simulink model "Full_model"  (R2019b)
settings: Solver=VariableStepAuto  StartTime=0.0  StopTime=150  RelTol=1e-3
model workspace: external: MATLAB File C:\Users\Techboard IITG\Downloads\Simscape4\Full_assem_DataFile.m (data not in the file)
undefined symbols (not defined in the file): _Default_sldprt, apx, ch_app, ch_cyc, cpz, L1, L2, L2rz, L2xf, L2yf, L2zf, l_app, max_avel, max_tvel, smiData, stand, TH1_ec_i, TH1_f, TH1_i, TH1_i_r, TH1_ri, TH2_ec_i, TH2_f, TH2_i, TH2_i_r, TH2_ri, TH3_f, TH3_i, TH3_ri, TH4_f, TH4_i, TH4_ri, time_ch_app, time_if, time_plug, time_ri, time_zchapp_down, time_zchapp_up, X, xp_dist, xp_vel, xpf_i, Y, yp_dist, yp_vel, ypf_i, Z, z_chapp, Z_i, zp_dist, zp_vel, zpf_i
libraries: simulink x68, fl_lib x36, sm_lib x22, nesl_utility x21, ee_lib x12
(part 2 of 3)

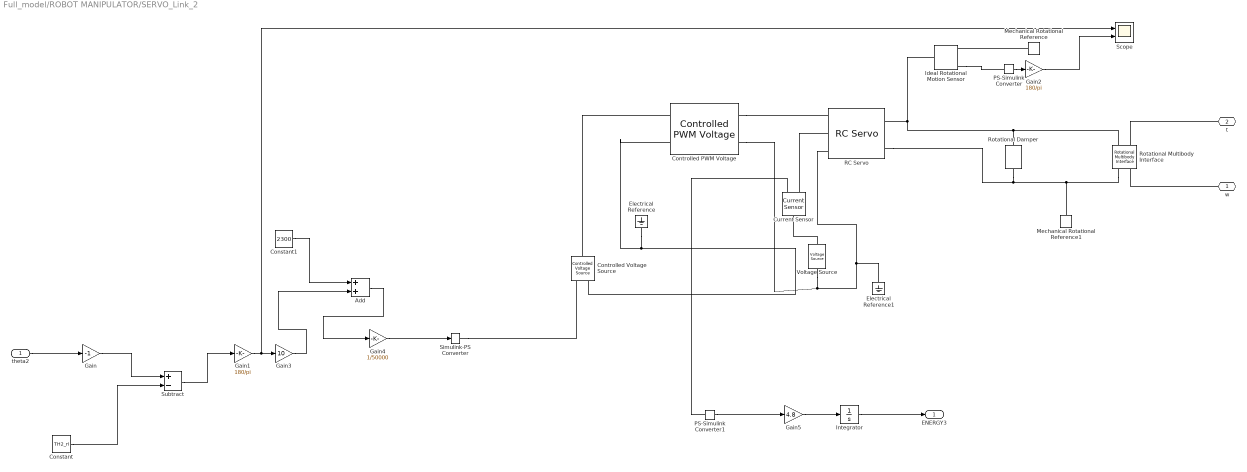
== system Full_model/ROBOT MANIPULATOR/SERVO_Link_2 ==
  theta2 : Inport
  Add : Sum
  Constant : Constant  Value=TH2_ri
  Constant1 : Constant  Value=2300
  Controlled PWM Voltage : ee_lib/Integrated Circuits/Controlled PWM Voltage  F=20 Hz  TD=0 s  pulse_width_offset=0 s  pulse_min=0 s  pwm_or_av=1  event_type=1  sample_time=1e-6 s  Vmin=0 V  Vmax=1 V  Vm=5 V  u_min=0  u_max=1
  Controlled Voltage Source : fl_lib/Electrical/Electrical Sources/Controlled Voltage Source
  Current Sensor : fl_lib/Electrical/Electrical Sensors/Current Sensor
      settings: SourceProductBaseCode=PW,SS,VE
  Electrical Reference : fl_lib/Electrical/Electrical Elements/Electrical Reference
  Electrical Reference1 : fl_lib/Electrical/Electrical Elements/Electrical Reference
  Gain : Gain  Gain=-1
  Gain1 : Gain  Gain=180/pi
  Gain2 : Gain  Gain=180/pi
  Gain3 : Gain  Gain=10
  Gain4 : Gain  Gain=1/50000
  Gain5 : Gain  Gain=4.8
  Ideal Rotational Motion Sensor : fl_lib/Mechanical/Mechanical Sensors/Ideal Rotational Motion Sensor  wrap_angle=simscape.enum.onoff.off  offset=0 rad
      settings: SourceProductBaseCode=PW,SS,VE
  Integrator : Integrator
  Mechanical Rotational Reference : fl_lib/Mechanical/Rotational Elements/Mechanical Rotational Reference
      settings: SourceProductBaseCode=PW,SS,VE
  Mechanical Rotational Reference1 : fl_lib/Mechanical/Rotational Elements/Mechanical Rotational Reference
  PS-Simulink Converter : nesl_utility/PS-Simulink Converter  PhysicalDomain=network_engine_domain  SubClassName=ps_output  LeftPortType=input  RightPortType=output  PseudoPeriodic=off  Frequencies=[]  VectorFormat=inherit  Unit=inherit  AffineConversion=off
      settings: SourceProductBaseCode=SS,PW,VE
  PS-Simulink Converter1 : nesl_utility/PS-Simulink Converter  PhysicalDomain=network_engine_domain  SubClassName=ps_output  LeftPortType=input  RightPortType=output  PseudoPeriodic=off  Frequencies=[]  VectorFormat=inherit  Unit=inherit  AffineConversion=off
      settings: SourceProductBaseCode=SS,PW,VE
  RC Servo : ee_lib/Electromechanical/Brushed Motors/RC Servo  stall_torque=25 kg*cm  time_60=0.28 s  nominal_voltage=4.8 V  rotational_range=[-90, 270] deg  pulse_width_range=[500, 4100] us  threshold=3 V  R_s=18 kOhm  resolution=0.1 deg  angle_meas_error=0 deg  backdrive_torque=0.5 kg*cm  ratio=320  inertia=0.01 g*cm^2  endstop_angles=[-90, 270] deg  endstop_stiffness=1e6 N*m/rad  endstop_damping=0.01 N*m/(rad/s)  enable_faults=0  fault_action=1  fault_type=1  enable_temporal_fault=0  t_fault=1 s  enable_behavioral_fault=0  max_permissible_current=1 A  t_fail_on_current=1 s  angle_specify=off  angle_priority=High  angle=90 deg  angle_nominal_specify=off  angle_nominal_unit=deg  angle_nominal_value=1  w_specify=off  w_priority=High  w=0 deg/s  w_nominal_specify=off  w_nominal_unit=deg/s  w_nominal_value=1  torque_specify=off  torque_priority=None  torque=0 N*m  torque_nominal_specify=off  torque_nominal_unit=N*m  torque_nominal_value=1  pulse_width_specify=off  pulse_width_priority=Low  pulse_width=1.5 ms  i_specify=off  i_priority=None  i=0 A  i_nominal_specify=off  i_nominal_unit=A  i_nominal_value=1  i_s_specify=off  i_s_priority=None  i_s=0 A  i_s_nominal_specify=off  i_s_nominal_unit=A  i_s_nominal_value=1  motor_torque_specify=off  motor_torque_priority=None  motor_torque=0 N*m  motor_torque_nominal_specify=off  motor_torque_nominal_unit=N*m  motor_torque_nominal_value=1  power_dissipated_specify=off  power_dissipated_priority=None  power_dissipated=0 W  power_dissipated_nominal_specify=off  power_dissipated_nominal_unit=W  power_dissipated_nominal_value=1  angle_demand_specify=off  angle_demand_priority=None  angle_demand=90 deg  angle_demand_nominal_specify=off  angle_demand_nominal_unit=deg  angle_demand_nominal_value=1  faulted_specify=off  faulted_priority=None  faulted=0  faulted_nominal_specify=off  faulted_nominal_unit=1  faulted_nominal_value=1
      settings: SourceProductBaseCode=PS  InternalSimscapePortConfiguration="{\"Bottom\":[],\"Left\":[{\"id\":\"s\",\"label\":\"s\",\"type\":\"foundation.electrical.electrical\"},{\"id\":\"p\",\"label\":\"+\",\"type\":\"foundation.electrical.electrical\"},{\"id\":\"n\",\"label\":\"-\",\"type\":\"foundation.electrical.electrical\"}],\"Right\":[{\"id\":\"R\",\"label\":\"R\",\"type\":\"foundation.mechanical.rotational.rotational\"},{\"id\":\"C\",\"label\":\"C\",\"type\":\"foundation.mechanical.rotational.rotational\"}],\"Top\":[]}"
  Rotational Damper : fl_lib/Mechanical/Rotational Elements/Rotational Damper  D=15 N*m*s/rad  w_specify=off  w_priority=None  w=0 rad/s  w_nominal_specify=off  w_nominal_unit=rad/s  w_nominal_value=1  t_specify=off  t_priority=None  t=0 N*m  t_nominal_specify=off  t_nominal_unit=N*m  t_nominal_value=1
      settings: SourceProductBaseCode=PW,SS,VE
  Rotational Multibody Interface : fl_lib/Mechanical/Multibody Interfaces/Rotational Multibody Interface
      settings: SourceProductBaseCode=PW,SS,VE
  Scope : Scope  NumInputPorts=2
  Simulink-PS Converter : nesl_utility/Simulink-PS Converter  PhysicalDomain=network_engine_domain  SubClassName=ps_input  LeftPortType=input  RightPortType=output  PseudoPeriodic=off  Frequencies=[]  NoiseDistribution=none  NoiseParameters=[]  Unit=1  AffineConversion=off  FilteringAndDerivatives=provide  SimscapeFilterOrder=1  InputFilterTimeConstant=0.001  UdotUserProvided=0
      settings: SourceProductBaseCode=PW,SS
  Subtract : Sum  Inputs=+-
  Voltage Source : ee_lib/Sources/Voltage Source  dc_voltage=4.8 V  ac_voltage=0 V  ac_shift=0 rad  ac_frequency=60 Hz  noise_mode=0  PSD=0 V^2/Hz  repeatability=1  auto_seed=2715962282  user_seed=0  sample_time=1e-3 s  i_specify=off  i_priority=None  i=0 A  i_nominal_specify=off  i_nominal_unit=A  i_nominal_value=1  v_specify=off  v_priority=None  v=0 V  v_nominal_specify=off  v_nominal_unit=V  v_nominal_value=1
  w : PMIOPort  Side=Right
  t : PMIOPort  Port=2  Side=Left
  ENERGY3 : Outport
  wires:
  Add/1 -> Gain4/1
  Gain4/1 -> Simulink-PS Converter/1
  Gain1/1 -> Scope/1, Gain3/1
  Gain3/1 -> Add/2
  Constant1/1 -> Add/1
  theta2/1 -> Gain/1
  PS-Simulink Converter/1 -> Gain2/1
  Gain/1 -> Subtract/1
  Constant/1 -> Subtract/2
  Subtract/1 -> Gain1/1
  PS-Simulink Converter1/1 -> Gain5/1
  Gain5/1 -> Integrator/1
  Integrator/1 -> ENERGY3/1
  Gain2/1 -> Scope/2
  connections:
  Rotational Damper/RConn1 -- Rotational Multibody Interface/RConn2 -- Mechanical Rotational Reference1/LConn1 -- RC Servo/RConn2
  Voltage Source/RConn1 -- Electrical Reference1/LConn1 -- RC Servo/LConn3 -- Controlled PWM Voltage/RConn2
  Electrical Reference/LConn1 -- Controlled Voltage Source/RConn2 -- Controlled PWM Voltage/LConn2
  Controlled Voltage Source/LConn1 -- Controlled PWM Voltage/LConn1
  Rotational Multibody Interface/LConn2 -- Rotational Damper/LConn1 -- Ideal Rotational Motion Sensor/LConn1 -- RC Servo/RConn1
  Controlled PWM Voltage/RConn1 -- RC Servo/LConn1
  Simulink-PS Converter/RConn1 -- Controlled Voltage Source/RConn1
  t/RConn1 -- Rotational Multibody Interface/LConn1
  Ideal Rotational Motion Sensor/RConn3 -- PS-Simulink Converter/LConn1
  Mechanical Rotational Reference/LConn1 -- Ideal Rotational Motion Sensor/RConn1
  w/RConn1 -- Rotational Multibody Interface/RConn1
  Voltage Source/LConn1 -- Current Sensor/LConn1
  Current Sensor/RConn2 -- RC Servo/LConn2
  Current Sensor/RConn1 -- PS-Simulink Converter1/LConn1

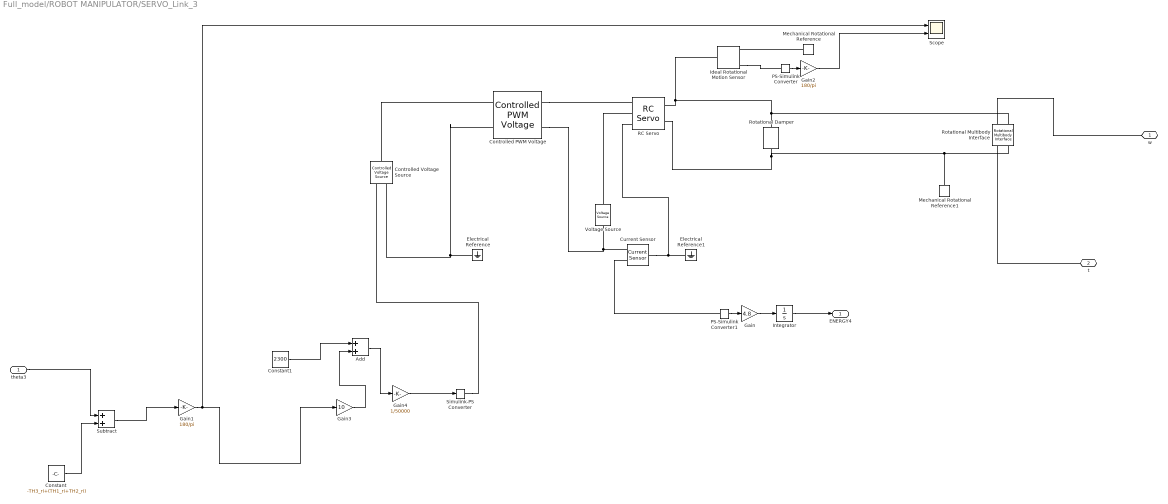
== system Full_model/ROBOT MANIPULATOR/SERVO_Link_3 ==
  theta3 : Inport
  Add : Sum
  Constant : Constant  Value=-TH3_ri+(TH1_ri+TH2_ri)
  Constant1 : Constant  Value=2300
  Controlled PWM Voltage : ee_lib/Integrated Circuits/Controlled PWM Voltage  F=20 Hz  TD=0 s  pulse_width_offset=0 s  pulse_min=0 s  pwm_or_av=1  event_type=1  sample_time=1e-6 s  Vmin=0 V  Vmax=1 V  Vm=5 V  u_min=0  u_max=1
  Controlled Voltage Source : fl_lib/Electrical/Electrical Sources/Controlled Voltage Source
  Current Sensor : fl_lib/Electrical/Electrical Sensors/Current Sensor
      settings: SourceProductBaseCode=PW,SS,VE
  Electrical Reference : fl_lib/Electrical/Electrical Elements/Electrical Reference
  Electrical Reference1 : fl_lib/Electrical/Electrical Elements/Electrical Reference
  Gain : Gain  Gain=4.8
  Gain1 : Gain  Gain=180/pi
  Gain2 : Gain  Gain=180/pi
  Gain3 : Gain  Gain=10
  Gain4 : Gain  Gain=1/50000
  Ideal Rotational Motion Sensor : fl_lib/Mechanical/Mechanical Sensors/Ideal Rotational Motion Sensor  wrap_angle=simscape.enum.onoff.off  offset=0 rad
      settings: SourceProductBaseCode=PW,SS,VE
  Integrator : Integrator
  Mechanical Rotational Reference : fl_lib/Mechanical/Rotational Elements/Mechanical Rotational Reference
      settings: SourceProductBaseCode=PW,SS,VE
  Mechanical Rotational Reference1 : fl_lib/Mechanical/Rotational Elements/Mechanical Rotational Reference
  PS-Simulink Converter : nesl_utility/PS-Simulink Converter  PhysicalDomain=network_engine_domain  SubClassName=ps_output  LeftPortType=input  RightPortType=output  PseudoPeriodic=off  Frequencies=[]  VectorFormat=inherit  Unit=inherit  AffineConversion=off
      settings: SourceProductBaseCode=SS,PW,VE
  PS-Simulink Converter1 : nesl_utility/PS-Simulink Converter  PhysicalDomain=network_engine_domain  SubClassName=ps_output  LeftPortType=input  RightPortType=output  PseudoPeriodic=off  Frequencies=[]  VectorFormat=inherit  Unit=inherit  AffineConversion=off
      settings: SourceProductBaseCode=SS,PW,VE
  RC Servo : ee_lib/Electromechanical/Brushed Motors/RC Servo  stall_torque=25 kg*cm  time_60=0.28 s  nominal_voltage=4.8 V  rotational_range=[-90,270] deg  pulse_width_range=[500, 4100] us  threshold=3 V  R_s=18 kOhm  resolution=0.1 deg  angle_meas_error=0 deg  backdrive_torque=0.5 kg*cm  ratio=320  inertia=0.01 g*cm^2  endstop_angles=[-90, 270] deg  endstop_stiffness=1e6 N*m/rad  endstop_damping=0.01 N*m/(rad/s)  enable_faults=0  fault_action=1  fault_type=1  enable_temporal_fault=0  t_fault=1 s  enable_behavioral_fault=0  max_permissible_current=1 A  t_fail_on_current=1 s  angle_specify=off  angle_priority=High  angle=90 deg  angle_nominal_specify=off  angle_nominal_unit=deg  angle_nominal_value=1  w_specify=off  w_priority=High  w=0 deg/s  w_nominal_specify=off  w_nominal_unit=deg/s  w_nominal_value=1  torque_specify=off  torque_priority=None  torque=0 N*m  torque_nominal_specify=off  torque_nominal_unit=N*m  torque_nominal_value=1  pulse_width_specify=off  pulse_width_priority=Low  pulse_width=1.5 ms  i_specify=off  i_priority=None  i=0 A  i_nominal_specify=off  i_nominal_unit=A  i_nominal_value=1  i_s_specify=off  i_s_priority=None  i_s=0 A  i_s_nominal_specify=off  i_s_nominal_unit=A  i_s_nominal_value=1  motor_torque_specify=off  motor_torque_priority=None  motor_torque=0 N*m  motor_torque_nominal_specify=off  motor_torque_nominal_unit=N*m  motor_torque_nominal_value=1  power_dissipated_specify=off  power_dissipated_priority=None  power_dissipated=0 W  power_dissipated_nominal_specify=off  power_dissipated_nominal_unit=W  power_dissipated_nominal_value=1  angle_demand_specify=off  angle_demand_priority=None  angle_demand=90 deg  angle_demand_nominal_specify=off  angle_demand_nominal_unit=deg  angle_demand_nominal_value=1  faulted_specify=off  faulted_priority=None  faulted=0  faulted_nominal_specify=off  faulted_nominal_unit=1  faulted_nominal_value=1
      settings: SourceProductBaseCode=PS  InternalSimscapePortConfiguration="{\"Bottom\":[],\"Left\":[{\"id\":\"s\",\"label\":\"s\",\"type\":\"foundation.electrical.electrical\"},{\"id\":\"p\",\"label\":\"+\",\"type\":\"foundation.electrical.electrical\"},{\"id\":\"n\",\"label\":\"-\",\"type\":\"foundation.electrical.electrical\"}],\"Right\":[{\"id\":\"R\",\"label\":\"R\",\"type\":\"foundation.mechanical.rotational.rotational\"},{\"id\":\"C\",\"label\":\"C\",\"type\":\"foundation.mechanical.rotational.rotational\"}],\"Top\":[]}"
  Rotational Damper : fl_lib/Mechanical/Rotational Elements/Rotational Damper  D=15 N*m*s/rad  w_specify=off  w_priority=None  w=0 rad/s  w_nominal_specify=off  w_nominal_unit=rad/s  w_nominal_value=1  t_specify=off  t_priority=None  t=0 N*m  t_nominal_specify=off  t_nominal_unit=N*m  t_nominal_value=1
      settings: SourceProductBaseCode=PW,SS,VE
  Rotational Multibody Interface : fl_lib/Mechanical/Multibody Interfaces/Rotational Multibody Interface
      settings: SourceProductBaseCode=PW,SS,VE
  Scope : Scope  NumInputPorts=2
  Simulink-PS Converter : nesl_utility/Simulink-PS Converter  PhysicalDomain=network_engine_domain  SubClassName=ps_input  LeftPortType=input  RightPortType=output  PseudoPeriodic=off  Frequencies=[]  NoiseDistribution=none  NoiseParameters=[]  Unit=1  AffineConversion=off  FilteringAndDerivatives=provide  SimscapeFilterOrder=1  InputFilterTimeConstant=0.001  UdotUserProvided=0
      settings: SourceProductBaseCode=PW,SS
  Subtract : Sum
  Voltage Source : ee_lib/Sources/Voltage Source  dc_voltage=4.8 V  ac_voltage=0 V  ac_shift=0 rad  ac_frequency=60 Hz  noise_mode=0  PSD=0 V^2/Hz  repeatability=1  auto_seed=418932850  user_seed=0  sample_time=1e-3 s  i_specify=off  i_priority=None  i=0 A  i_nominal_specify=off  i_nominal_unit=A  i_nominal_value=1  v_specify=off  v_priority=None  v=0 V  v_nominal_specify=off  v_nominal_unit=V  v_nominal_value=1
  w : PMIOPort  Side=Right
  t : PMIOPort  Port=2  Side=Left
  ENERGY4 : Outport
  wires:
  Add/1 -> Gain4/1
  Gain4/1 -> Simulink-PS Converter/1
  Gain3/1 -> Add/2
  Constant1/1 -> Add/1
  PS-Simulink Converter/1 -> Gain2/1
  theta3/1 -> Subtract/1
  Gain1/1 -> Scope/1, Gain3/1
  Constant/1 -> Subtract/2
  Subtract/1 -> Gain1/1
  Gain2/1 -> Scope/2
  PS-Simulink Converter1/1 -> Gain/1
  Gain/1 -> Integrator/1
  Integrator/1 -> ENERGY4/1
  connections:
  Rotational Damper/RConn1 -- RC Servo/RConn2 -- Mechanical Rotational Reference1/LConn1 -- Rotational Multibody Interface/LConn2
  Rotational Multibody Interface/RConn1 -- w/RConn1
  Electrical Reference1/LConn1 -- Current Sensor/LConn1 -- RC Servo/LConn3
  Electrical Reference/LConn1 -- Controlled PWM Voltage/LConn2 -- Controlled Voltage Source/RConn2
  Controlled Voltage Source/LConn1 -- Controlled PWM Voltage/LConn1
  Rotational Damper/LConn1 -- Ideal Rotational Motion Sensor/LConn1 -- RC Servo/RConn1 -- Rotational Multibody Interface/RConn2
  Voltage Source/LConn1 -- RC Servo/LConn2
  Controlled PWM Voltage/RConn1 -- RC Servo/LConn1
  Simulink-PS Converter/RConn1 -- Controlled Voltage Source/RConn1
  t/RConn1 -- Rotational Multibody Interface/LConn1
  Ideal Rotational Motion Sensor/RConn3 -- PS-Simulink Converter/LConn1
  Mechanical Rotational Reference/LConn1 -- Ideal Rotational Motion Sensor/RConn1
  Controlled PWM Voltage/RConn2 -- Current Sensor/RConn2 -- Voltage Source/RConn1
  Current Sensor/RConn1 -- PS-Simulink Converter1/LConn1

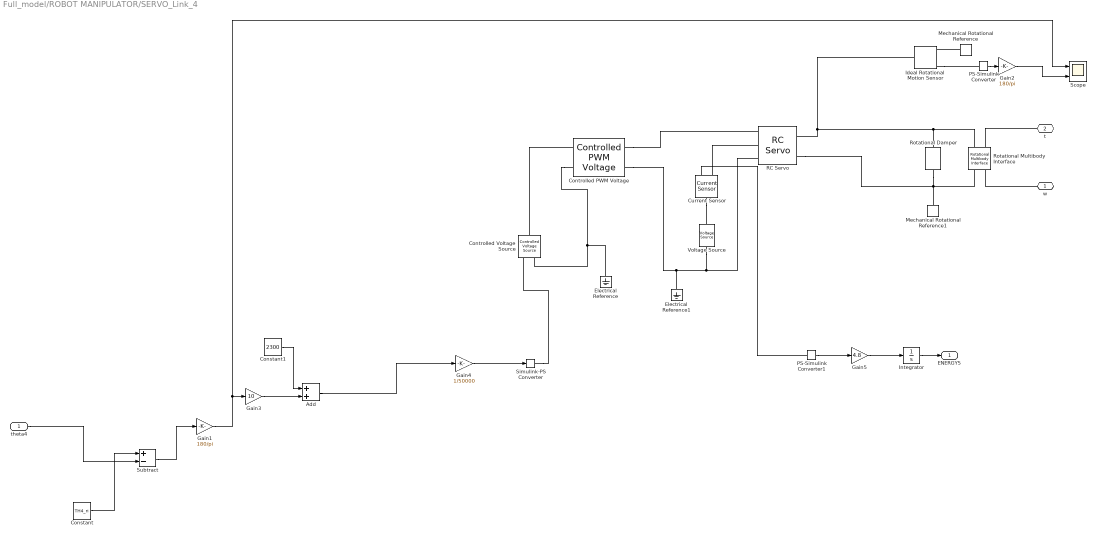
== system Full_model/ROBOT MANIPULATOR/SERVO_Link_4 ==
  theta4 : Inport
  Add : Sum
  Constant : Constant  Value=TH4_ri
  Constant1 : Constant  Value=2300
  Controlled PWM Voltage : ee_lib/Integrated Circuits/Controlled PWM Voltage  F=20 Hz  TD=0 s  pulse_width_offset=0 s  pulse_min=0 s  pwm_or_av=1  event_type=1  sample_time=1e-6 s  Vmin=0 V  Vmax=1 V  Vm=5 V  u_min=0  u_max=1
  Controlled Voltage Source : fl_lib/Electrical/Electrical Sources/Controlled Voltage Source
  Current Sensor : fl_lib/Electrical/Electrical Sensors/Current Sensor
      settings: SourceProductBaseCode=PW,SS,VE
  Electrical Reference : fl_lib/Electrical/Electrical Elements/Electrical Reference
  Electrical Reference1 : fl_lib/Electrical/Electrical Elements/Electrical Reference
  Gain1 : Gain  Gain=180/pi
  Gain2 : Gain  Gain=180/pi
  Gain3 : Gain  Gain=10
  Gain4 : Gain  Gain=1/50000
  Gain5 : Gain  Gain=4.8
  Ideal Rotational Motion Sensor : fl_lib/Mechanical/Mechanical Sensors/Ideal Rotational Motion Sensor  wrap_angle=simscape.enum.onoff.off  offset=0 rad
      settings: SourceProductBaseCode=PW,SS,VE
  Integrator : Integrator
  Mechanical Rotational Reference : fl_lib/Mechanical/Rotational Elements/Mechanical Rotational Reference
      settings: SourceProductBaseCode=PW,SS,VE
  Mechanical Rotational Reference1 : fl_lib/Mechanical/Rotational Elements/Mechanical Rotational Reference
  PS-Simulink Converter : nesl_utility/PS-Simulink Converter  PhysicalDomain=network_engine_domain  SubClassName=ps_output  LeftPortType=input  RightPortType=output  PseudoPeriodic=off  Frequencies=[]  VectorFormat=inherit  Unit=inherit  AffineConversion=off
      settings: SourceProductBaseCode=SS,PW,VE
  PS-Simulink Converter1 : nesl_utility/PS-Simulink Converter  PhysicalDomain=network_engine_domain  SubClassName=ps_output  LeftPortType=input  RightPortType=output  PseudoPeriodic=off  Frequencies=[]  VectorFormat=inherit  Unit=inherit  AffineConversion=off
      settings: SourceProductBaseCode=SS,PW,VE
  RC Servo : ee_lib/Electromechanical/Brushed Motors/RC Servo  stall_torque=25 kg*cm  time_60=0.28 s  nominal_voltage=4.8 V  rotational_range=[-90, 270] deg  pulse_width_range=[500, 4100] us  threshold=3 V  R_s=18 kOhm  resolution=0.1 deg  angle_meas_error=0 deg  backdrive_torque=0.5 kg*cm  ratio=320  inertia=0.01 g*cm^2  endstop_angles=[-90, 270] deg  endstop_stiffness=1e6 N*m/rad  endstop_damping=0.01 N*m/(rad/s)  enable_faults=0  fault_action=1  fault_type=1  enable_temporal_fault=0  t_fault=1 s  enable_behavioral_fault=0  max_permissible_current=1 A  t_fail_on_current=1 s  angle_specify=off  angle_priority=None  angle=5 deg  angle_nominal_specify=off  angle_nominal_unit=deg  angle_nominal_value=1  w_specify=off  w_priority=High  w=0 deg/s  w_nominal_specify=off  w_nominal_unit=deg/s  w_nominal_value=1  torque_specify=off  torque_priority=None  torque=0 N*m  torque_nominal_specify=off  torque_nominal_unit=N*m  torque_nominal_value=1  pulse_width_specify=off  pulse_width_priority=High  pulse_width=2 ms  i_specify=off  i_priority=None  i=0 A  i_nominal_specify=off  i_nominal_unit=A  i_nominal_value=1  i_s_specify=off  i_s_priority=None  i_s=0 A  i_s_nominal_specify=off  i_s_nominal_unit=A  i_s_nominal_value=1  motor_torque_specify=off  motor_torque_priority=None  motor_torque=0 N*m  motor_torque_nominal_specify=off  motor_torque_nominal_unit=N*m  motor_torque_nominal_value=1  power_dissipated_specify=off  power_dissipated_priority=None  power_dissipated=0 W  power_dissipated_nominal_specify=off  power_dissipated_nominal_unit=W  power_dissipated_nominal_value=1  angle_demand_specify=off  angle_demand_priority=None  angle_demand=90 deg  angle_demand_nominal_specify=off  angle_demand_nominal_unit=deg  angle_demand_nominal_value=1  faulted_specify=off  faulted_priority=None  faulted=0  faulted_nominal_specify=off  faulted_nominal_unit=1  faulted_nominal_value=1
      settings: SourceProductBaseCode=PS  InternalSimscapePortConfiguration="{\"Bottom\":[],\"Left\":[{\"id\":\"s\",\"label\":\"s\",\"type\":\"foundation.electrical.electrical\"},{\"id\":\"p\",\"label\":\"+\",\"type\":\"foundation.electrical.electrical\"},{\"id\":\"n\",\"label\":\"-\",\"type\":\"foundation.electrical.electrical\"}],\"Right\":[{\"id\":\"R\",\"label\":\"R\",\"type\":\"foundation.mechanical.rotational.rotational\"},{\"id\":\"C\",\"label\":\"C\",\"type\":\"foundation.mechanical.rotational.rotational\"}],\"Top\":[]}"
  Rotational Damper : fl_lib/Mechanical/Rotational Elements/Rotational Damper  D=15 N*m*s/rad  w_specify=off  w_priority=None  w=0 rad/s  w_nominal_specify=off  w_nominal_unit=rad/s  w_nominal_value=1  t_specify=off  t_priority=None  t=0 N*m  t_nominal_specify=off  t_nominal_unit=N*m  t_nominal_value=1
      settings: SourceProductBaseCode=PW,SS,VE
  Rotational Multibody Interface : fl_lib/Mechanical/Multibody Interfaces/Rotational Multibody Interface
      settings: SourceProductBaseCode=PW,SS,VE
  Scope : Scope  NumInputPorts=2
  Simulink-PS Converter : nesl_utility/Simulink-PS Converter  PhysicalDomain=network_engine_domain  SubClassName=ps_input  LeftPortType=input  RightPortType=output  PseudoPeriodic=off  Frequencies=[]  NoiseDistribution=none  NoiseParameters=[]  Unit=1  AffineConversion=off  FilteringAndDerivatives=provide  SimscapeFilterOrder=1  InputFilterTimeConstant=0.001  UdotUserProvided=0
      settings: SourceProductBaseCode=PW,SS
  Subtract : Sum  Inputs=+-
  Voltage Source : ee_lib/Sources/Voltage Source  dc_voltage=4.8 V  ac_voltage=0 V  ac_shift=0 rad  ac_frequency=60 Hz  noise_mode=0  PSD=0 V^2/Hz  repeatability=1  auto_seed=2348838240  user_seed=0  sample_time=1e-3 s  i_specify=off  i_priority=None  i=0 A  i_nominal_specify=off  i_nominal_unit=A  i_nominal_value=1  v_specify=off  v_priority=None  v=0 V  v_nominal_specify=off  v_nominal_unit=V  v_nominal_value=1
  w : PMIOPort  Side=Right
  t : PMIOPort  Port=2  Side=Left
  ENERGY5 : Outport
  wires:
  Add/1 -> Gain4/1
  Gain4/1 -> Simulink-PS Converter/1
  Gain1/1 -> Scope/1, Gain3/1
  Gain3/1 -> Add/2
  Constant1/1 -> Add/1
  PS-Simulink Converter/1 -> Gain2/1
  Subtract/1 -> Gain1/1
  PS-Simulink Converter1/1 -> Gain5/1
  Gain5/1 -> Integrator/1
  Integrator/1 -> ENERGY5/1
  theta4/1 -> Subtract/2
  Constant/1 -> Subtract/1
  Gain2/1 -> Scope/2
  connections:
  RC Servo/RConn2 -- Rotational Multibody Interface/RConn2 -- Mechanical Rotational Reference1/LConn1 -- Rotational Damper/RConn1
  Voltage Source/RConn1 -- Electrical Reference1/LConn1 -- Controlled PWM Voltage/RConn2 -- RC Servo/LConn3
  Controlled PWM Voltage/LConn2 -- Electrical Reference/LConn1 -- Controlled Voltage Source/RConn2
  Controlled Voltage Source/LConn1 -- Controlled PWM Voltage/LConn1
  Rotational Damper/LConn1 -- Ideal Rotational Motion Sensor/LConn1 -- RC Servo/RConn1 -- Rotational Multibody Interface/LConn2
  Controlled PWM Voltage/RConn1 -- RC Servo/LConn1
  Simulink-PS Converter/RConn1 -- Controlled Voltage Source/RConn1
  t/RConn1 -- Rotational Multibody Interface/LConn1
  Mechanical Rotational Reference/LConn1 -- Ideal Rotational Motion Sensor/RConn1
  Ideal Rotational Motion Sensor/RConn3 -- PS-Simulink Converter/LConn1
  w/RConn1 -- Rotational Multibody Interface/RConn1
  Current Sensor/LConn1 -- Voltage Source/LConn1
  Current Sensor/RConn2 -- RC Servo/LConn2
  Current Sensor/RConn1 -- PS-Simulink Converter1/LConn1

== system Full_model/TRAJECTORY_PLANNING/CHAPP_INTER1 ==
  TH_i : Inport
  TH : Inport  Port=2
  MATLAB Function12 : MATLAB Function  TreatAsAtomicUnit=on
  Saturation Dynamic10 : simulink/Discontinuities/Saturation Dynamic  OutMin=[]  OutMax=[]  OutDataTypeStr=Inherit: Same as second input  OutDataType=fixdt(1, 16)  OutScaling=2^-10  DoSatur=off
  Switch14 : Switch  Criteria=u2 > Threshold
  r_neg10 : simulink/Sources/Ramp  slope=-max_avel  start=(time_ri+time_zchapp_up)  InitialOutput=0
  r_pos10 : simulink/Sources/Ramp  slope=max_avel  start=(time_ri+time_zchapp_up)  InitialOutput=0
  y : Outport
  wires:
  TH_i/1 -> MATLAB Function12/1(TH_i)
  MATLAB Function12/3(l) -> Saturation Dynamic10/3
  Saturation Dynamic10/1 -> y/1
  TH/1 -> MATLAB Function12/2(TH)
  r_pos10/1 -> Switch14/1
  MATLAB Function12/2(y) -> Switch14/2
  Switch14/1 -> Saturation Dynamic10/2
  r_neg10/1 -> Switch14/3
  MATLAB Function12/1(u) -> Saturation Dynamic10/1

== system Full_model/TRAJECTORY_PLANNING/CHAPP_INTER2 ==
  TH : Inport
  TH_i : Inport  Port=2
  MATLAB Function13 : MATLAB Function  TreatAsAtomicUnit=on
  Saturation Dynamic11 : simulink/Discontinuities/Saturation Dynamic  OutMin=[]  OutMax=[]  OutDataTypeStr=Inherit: Same as second input  OutDataType=fixdt(1, 16)  OutScaling=2^-10  DoSatur=off
  Switch15 : Switch  Criteria=u2 > Threshold
  r_neg11 : simulink/Sources/Ramp  slope=-max_avel  start=(time_ri+time_zchapp_up)  InitialOutput=0
  r_pos11 : simulink/Sources/Ramp  slope=max_avel  start=(time_ri+time_zchapp_up)  InitialOutput=0
  y : Outport
  wires:
  Saturation Dynamic11/1 -> y/1
  MATLAB Function13/1(u) -> Saturation Dynamic11/1
  r_neg11/1 -> Switch15/3
  r_pos11/1 -> Switch15/1
  TH_i/1 -> MATLAB Function13/2(TH_i)
  TH/1 -> MATLAB Function13/1(TH)
  MATLAB Function13/2(y) -> Switch15/2
  Switch15/1 -> Saturation Dynamic11/2
  MATLAB Function13/3(l) -> Saturation Dynamic11/3

== system Full_model/TRAJECTORY_PLANNING/CHK_CHAPP1 ==
  In1 : Inport
  Constant46 : Constant  Value=ch_app
  Constant49 : Constant  Value=0
  Switch19 : Switch  Criteria=u2 > Threshold
  Out1 : Outport
  wires:
  Switch19/1 -> Out1/1
  In1/1 -> Switch19/1
  Constant49/1 -> Switch19/3
  Constant46/1 -> Switch19/2

== system Full_model/TRAJECTORY_PLANNING/CHK_CHAPP2 ==
  In1 : Inport
  Constant47 : Constant  Value=ch_app
  Constant48 : Constant  Value=0
  Switch13 : Switch  Criteria=u2 > Threshold
  Out1 : Outport
  wires:
  Switch13/1 -> Out1/1
  In1/1 -> Switch13/1
  Constant48/1 -> Switch13/3
  Constant47/1 -> Switch13/2

== system Full_model/TRAJECTORY_PLANNING/IF_INTER1 ==
  note: set waypt. theta1
  TH_i : Inport
  TH : Inport  Port=2
  MATLAB Function14 : MATLAB Function  TreatAsAtomicUnit=on
  Saturation Dynamic12 : simulink/Discontinuities/Saturation Dynamic  OutMin=[]  OutMax=[]  OutDataTypeStr=Inherit: Same as second input  OutDataType=fixdt(1, 16)  OutScaling=2^-10  DoSatur=off
  Switch16 : Switch  Criteria=u2 > Threshold
  r_neg12 : simulink/Sources/Ramp  slope=-max_avel  start=(time_ri+time_ch_app)  InitialOutput=0
  r_pos12 : simulink/Sources/Ramp  slope=max_avel  start=(time_ri+time_ch_app)  InitialOutput=0
  y : Outport
  wires:
  MATLAB Function14/3(l) -> Saturation Dynamic12/3
  MATLAB Function14/2(y) -> Switch16/2
  MATLAB Function14/1(u) -> Saturation Dynamic12/1
  Switch16/1 -> Saturation Dynamic12/2
  r_neg12/1 -> Switch16/3
  Saturation Dynamic12/1 -> y/1
  r_pos12/1 -> Switch16/1
  TH/1 -> MATLAB Function14/2(TH)
  TH_i/1 -> MATLAB Function14/1(TH_i)

== system Full_model/TRAJECTORY_PLANNING/IF_INTER2 ==
  TH : Inport
  TH_i : Inport  Port=2
  MATLAB Function15 : MATLAB Function  TreatAsAtomicUnit=on
  Saturation Dynamic13 : simulink/Discontinuities/Saturation Dynamic  OutMin=[]  OutMax=[]  OutDataTypeStr=Inherit: Same as second input  OutDataType=fixdt(1, 16)  OutScaling=2^-10  DoSatur=off
  Switch17 : Switch  Criteria=u2 > Threshold
  r_neg13 : simulink/Sources/Ramp  slope=-max_avel  start=(time_ri+time_ch_app)  InitialOutput=0
  r_pos13 : simulink/Sources/Ramp  slope=max_avel  start=(time_ri+time_ch_app)  InitialOutput=0
  y : Outport
  wires:
  TH_i/1 -> MATLAB Function15/2(TH_i)
  Saturation Dynamic13/1 -> y/1
  r_neg13/1 -> Switch17/3
  r_pos13/1 -> Switch17/1
  MATLAB Function15/3(l) -> Saturation Dynamic13/3
  TH/1 -> MATLAB Function15/1(TH)
  MATLAB Function15/1(u) -> Saturation Dynamic13/1
  Switch17/1 -> Saturation Dynamic13/2
  MATLAB Function15/2(y) -> Switch17/2

== system Full_model/TRAJECTORY_PLANNING/IF_INTER3 ==
  note: set waypt. theta1
  TH_i : Inport
  TH : Inport  Port=2
  MATLAB Function14 : MATLAB Function  TreatAsAtomicUnit=on
  Saturation Dynamic12 : simulink/Discontinuities/Saturation Dynamic  OutMin=[]  OutMax=[]  OutDataTypeStr=Inherit: Same as second input  OutDataType=fixdt(1, 16)  OutScaling=2^-10  DoSatur=off
  Switch16 : Switch  Criteria=u2 > Threshold
  r_neg12 : simulink/Sources/Ramp  slope=-max_avel  start=(time_ri+time_ch_app+time_if+(2*time_plug)+ch_cyc)  InitialOutput=0
  r_pos12 : simulink/Sources/Ramp  slope=max_avel  start=(time_ri+time_ch_app+time_if+(2*time_plug)+ch_cyc)  InitialOutput=0
  y : Outport
  wires:
  MATLAB Function14/3(l) -> Saturation Dynamic12/3
  MATLAB Function14/2(y) -> Switch16/2
  MATLAB Function14/1(u) -> Saturation Dynamic12/1
  Switch16/1 -> Saturation Dynamic12/2
  r_neg12/1 -> Switch16/3
  Saturation Dynamic12/1 -> y/1
  r_pos12/1 -> Switch16/1
  TH/1 -> MATLAB Function14/2(TH)
  TH_i/1 -> MATLAB Function14/1(TH_i)

== system Full_model/TRAJECTORY_PLANNING/IF_INTER4 ==
  TH : Inport
  TH_i : Inport  Port=2
  MATLAB Function15 : MATLAB Function  TreatAsAtomicUnit=on
  Saturation Dynamic13 : simulink/Discontinuities/Saturation Dynamic  OutMin=[]  OutMax=[]  OutDataTypeStr=Inherit: Same as second input  OutDataType=fixdt(1, 16)  OutScaling=2^-10  DoSatur=off
  Switch17 : Switch  Criteria=u2 > Threshold
  r_neg13 : simulink/Sources/Ramp  slope=-max_avel  start=(time_ri+time_ch_app+time_if+(2*time_plug)+ch_cyc)  InitialOutput=0
  r_pos13 : simulink/Sources/Ramp  slope=max_avel  start=(time_ri+time_ch_app+time_if+(2*time_plug)+ch_cyc)  InitialOutput=0
  y : Outport
  wires:
  TH_i/1 -> MATLAB Function15/2(TH_i)
  Saturation Dynamic13/1 -> y/1
  r_neg13/1 -> Switch17/3
  r_pos13/1 -> Switch17/1
  MATLAB Function15/3(l) -> Saturation Dynamic13/3
  TH/1 -> MATLAB Function15/1(TH)
  MATLAB Function15/1(u) -> Saturation Dynamic13/1
  Switch17/1 -> Saturation Dynamic13/2
  MATLAB Function15/2(y) -> Switch17/2

== system Full_model/TRAJECTORY_PLANNING/Subsystem ==
  TH_i : Inport
  TH : Inport  Port=2
  MATLAB Function10 : MATLAB Function  TreatAsAtomicUnit=on
  Saturation Dynamic8 : simulink/Discontinuities/Saturation Dynamic  OutMin=[]  OutMax=[]  OutDataTypeStr=Inherit: Same as second input  OutDataType=fixdt(1, 16)  OutScaling=2^-10  DoSatur=off
  Switch11 : Switch  Criteria=u2 > Threshold
  r_neg8 : simulink/Sources/Ramp  slope=-max_avel  start=0  InitialOutput=TH1_ri
  r_pos8 : simulink/Sources/Ramp  slope=max_avel  start=0  InitialOutput=TH1_ri
  y : Outport
  wires:
  TH_i/1 -> MATLAB Function10/1(TH_i)
  r_pos8/1 -> Switch11/1
  r_neg8/1 -> Switch11/3
  Saturation Dynamic8/1 -> y/1
  MATLAB Function10/2(y) -> Switch11/2
  MATLAB Function10/1(u) -> Saturation Dynamic8/1
  MATLAB Function10/3(l) -> Saturation Dynamic8/3
  Switch11/1 -> Saturation Dynamic8/2
  TH/1 -> MATLAB Function10/2(TH)

== system Full_model/TRAJECTORY_PLANNING/Subsystem1 ==
  TH : Inport
  TH_i : Inport  Port=2
  MATLAB Function11 : MATLAB Function  TreatAsAtomicUnit=on
  Saturation Dynamic9 : simulink/Discontinuities/Saturation Dynamic  OutMin=[]  OutMax=[]  OutDataTypeStr=Inherit: Same as second input  OutDataType=fixdt(1, 16)  OutScaling=2^-10  DoSatur=off
  Switch12 : Switch  Criteria=u2 > Threshold
  r_neg9 : simulink/Sources/Ramp  slope=-max_avel  start=0  InitialOutput=TH2_ri
  r_pos9 : simulink/Sources/Ramp  slope=max_avel  start=0  InitialOutput=TH2_ri
  y : Outport
  wires:
  Saturation Dynamic9/1 -> y/1
  MATLAB Function11/2(y) -> Switch12/2
  MATLAB Function11/1(u) -> Saturation Dynamic9/1
  TH/1 -> MATLAB Function11/1(TH)
  TH_i/1 -> MATLAB Function11/2(TH_i)
  Switch12/1 -> Saturation Dynamic9/2
  r_pos9/1 -> Switch12/1
  MATLAB Function11/3(l) -> Saturation Dynamic9/3
  r_neg9/1 -> Switch12/3

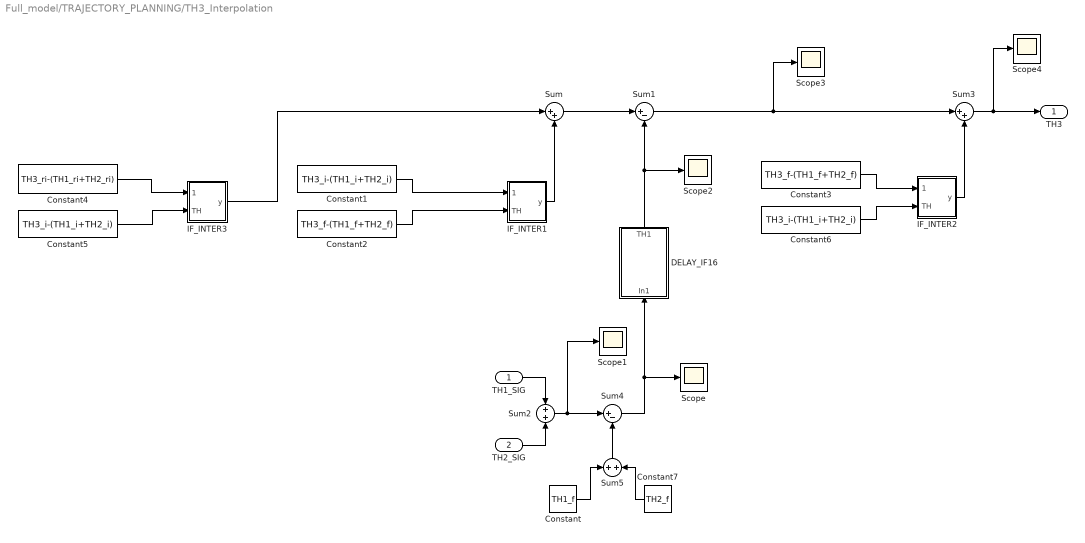
== system Full_model/TRAJECTORY_PLANNING/TH3_Interpolation ==
  TH1_SIG : Inport
  TH2_SIG : Inport  Port=2
  Constant : Constant  Value=TH1_f
  Constant1 : Constant  Value=TH3_i-(TH1_i+TH2_i)
  Constant2 : Constant  Value=TH3_f-(TH1_f+TH2_f)
  Constant3 : Constant  Value=TH3_f-(TH1_f+TH2_f)
  Constant4 : Constant  Value=TH3_ri-(TH1_ri+TH2_ri)
  Constant5 : Constant  Value=TH3_i-(TH1_i+TH2_i)
  Constant6 : Constant  Value=TH3_i-(TH1_i+TH2_i)
  Constant7 : Constant  Value=TH2_f
  DELAY_IF16 : Subsystem
  IF_INTER1 : Subsystem
  IF_INTER2 : Subsystem
  IF_INTER3 : Subsystem
  Scope{,1..4} (5 alike) : Scope
  Sum : Sum  Inputs=|++
  Sum1 : Sum  Inputs=|+-
  Sum2 : Sum
  Sum3 : Sum  Inputs=|++
  Sum4 : Sum  Inputs=|+-
  Sum5 : Sum
  TH3 : Outport
  wires:
  DELAY_IF16/1(TH1) -> Sum1/2, Scope2/1
  Sum4/1 -> DELAY_IF16/1(In1), Scope/1
  Sum5/1 -> Sum4/2
  Constant7/1 -> Sum5/2
  Constant/1 -> Sum5/1
  Sum2/1 -> Sum4/1, Scope1/1
  Sum3/1 -> TH3/1, Scope4/1
  Sum1/1 -> Sum3/1, Scope3/1
  IF_INTER2/1(y) -> Sum3/2
  Constant6/1 -> IF_INTER2/2(TH)
  Constant3/1 -> IF_INTER2/1(TH_i)
  TH2_SIG/1 -> Sum2/2
  TH1_SIG/1 -> Sum2/1
  Constant1/1 -> IF_INTER1/1(TH_i)
  Constant2/1 -> IF_INTER1/2(TH)
  IF_INTER1/1(y) -> Sum/2
  IF_INTER3/1(y) -> Sum/1
  Constant5/1 -> IF_INTER3/2(TH)
  Constant4/1 -> IF_INTER3/1(TH_i)
  Sum/1 -> Sum1/1

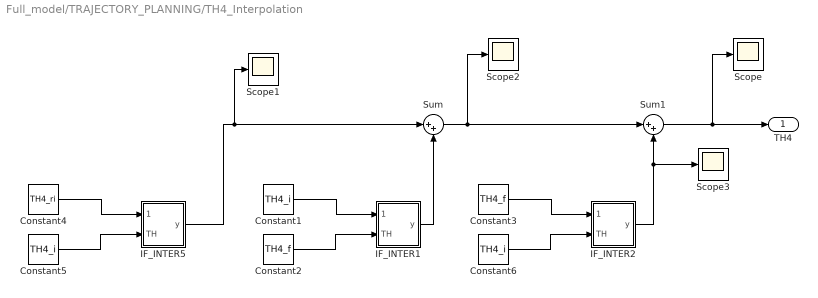
== system Full_model/TRAJECTORY_PLANNING/TH4_Interpolation ==
  Constant1 : Constant  Value=TH4_i
  Constant2 : Constant  Value=TH4_f
  Constant3 : Constant  Value=TH4_f
  Constant4 : Constant  Value=TH4_ri
  Constant5 : Constant  Value=TH4_i
  Constant6 : Constant  Value=TH4_i
  IF_INTER1 : Subsystem
  IF_INTER2 : Subsystem
  IF_INTER5 : Subsystem
  Scope{,1..3} (4 alike) : Scope
  Sum : Sum  Inputs=|++
  Sum1 : Sum  Inputs=|++
  TH4 : Outport
  wires:
  Sum/1 -> Sum1/1, Scope2/1
  Sum1/1 -> TH4/1, Scope/1
  Constant6/1 -> IF_INTER2/2(TH)
  Constant3/1 -> IF_INTER2/1(TH_i)
  IF_INTER2/1(y) -> Sum1/2, Scope3/1
  IF_INTER1/1(y) -> Sum/2
  IF_INTER5/1(y) -> Sum/1, Scope1/1
  Constant1/1 -> IF_INTER1/1(TH_i)
  Constant2/1 -> IF_INTER1/2(TH)
  Constant5/1 -> IF_INTER5/2(TH)
  Constant4/1 -> IF_INTER5/1(TH_i)

== system Full_model/TRAJECTORY_PLANNING/TS_JA_Interpolation ==
  Constant13 : Constant  Value=TH2_f
  Constant14 : Constant  Value=TH1_f
  DELAY_IF16 : Subsystem
  DELAY_IF17 : Subsystem
  IK_BLOCK1 : Subsystem
  Sum17 : Sum  Inputs=-+|
  Sum22 : Sum  Inputs=|+-
  X_Plug-in_TS_Interpolation : Subsystem
  Y_Plug-in_TS_Interpolation : Subsystem
  TH1 : Outport
  TH2 : Outport  Port=2
  wires:
  DELAY_IF17/1(TH2) -> TH2/1
  IK_BLOCK1/1(TH1) -> Sum17/2
  Constant13/1 -> Sum22/2
  Sum22/1 -> DELAY_IF17/1(In1)
  Constant14/1 -> Sum17/1
  DELAY_IF16/1(TH1) -> TH1/1
  IK_BLOCK1/2(TH2) -> Sum22/1
  Sum17/1 -> DELAY_IF16/1(In1)
  Y_Plug-in_TS_Interpolation/1(Y_TS) -> IK_BLOCK1/2(YE)
  X_Plug-in_TS_Interpolation/1(X_TS) -> IK_BLOCK1/1(XE)

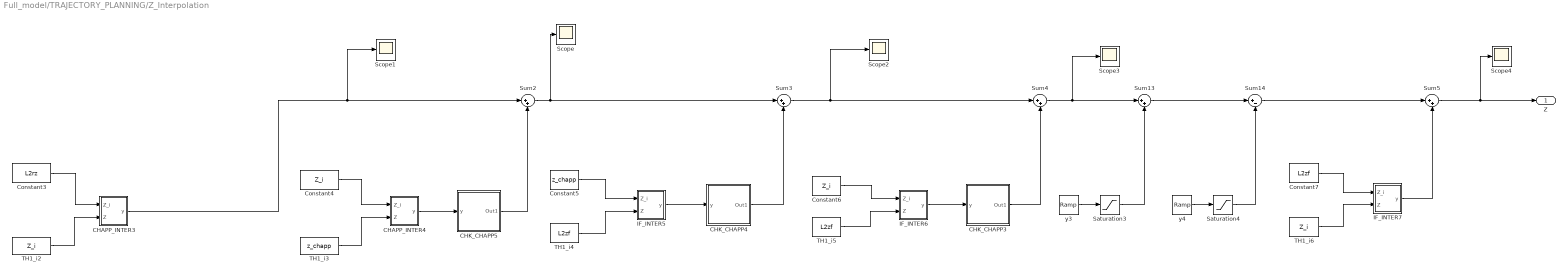
== system Full_model/TRAJECTORY_PLANNING/Z_Interpolation ==
  CHAPP_INTER3 : Subsystem
  CHAPP_INTER4 : Subsystem
  CHK_CHAPP3 : Subsystem
  CHK_CHAPP4 : Subsystem
  CHK_CHAPP5 : Subsystem
  Constant3 : Constant  Value=L2rz
  Constant4 : Constant  Value=Z_i
  Constant5 : Constant  Value=z_chapp
  Constant6 : Constant  Value=Z_i
  Constant7 : Constant  Value=L2zf
  IF_INTER5 : Subsystem
  IF_INTER6 : Subsystem
  IF_INTER7 : Subsystem
  Saturation3 : Saturate  UpperLimit=max(zp_dist,-zp_dist)  LowerLimit=min(zp_dist,-zp_dist)
  Saturation4 : Saturate  UpperLimit=max(zp_dist,-zp_dist)  LowerLimit=min(zp_dist,-zp_dist)
  Scope{,1..4} (5 alike) : Scope
  Sum{2..5,13} (5 alike) : Sum  Inputs=|++
  Sum14 : Sum  Inputs=|+-
  TH1_i2 : Constant  Value=Z_i
  TH1_i3 : Constant  Value=z_chapp
  TH1_i4 : Constant  Value=L2zf
  TH1_i5 : Constant  Value=L2zf
  TH1_i6 : Constant  Value=Z_i
  y3 : simulink/Sources/Ramp  slope=zp_vel  start=(time_ri+time_ch_app+time_if)  InitialOutput=0
  y4 : simulink/Sources/Ramp  slope=zp_vel  start=(time_ri+time_ch_app+time_if+(time_plug)+ch_cyc)  InitialOutput=0
  Z : Outport
  wires:
  TH1_i5/1 -> IF_INTER6/2(Z)
  y4/1 -> Saturation4/1
  Constant3/1 -> CHAPP_INTER3/1(Z_i)
  Saturation3/1 -> Sum13/2
  TH1_i3/1 -> CHAPP_INTER4/2(Z)
  CHK_CHAPP3/1(Out1) -> Sum4/2
  TH1_i4/1 -> IF_INTER5/2(Z)
  CHK_CHAPP5/1(Out1) -> Sum2/2
  Sum2/1 -> Sum3/1, Scope/1
  CHAPP_INTER4/1(y) -> CHK_CHAPP5/1(y)
  IF_INTER5/1(y) -> CHK_CHAPP4/1(y)
  CHK_CHAPP4/1(Out1) -> Sum3/2
  Sum5/1 -> Z/1, Scope4/1
  TH1_i6/1 -> IF_INTER7/2(Z)
  IF_INTER7/1(y) -> Sum5/2
  Sum3/1 -> Sum4/1, Scope2/1
  Saturation4/1 -> Sum14/2
  Sum4/1 -> Sum13/1, Scope3/1
  Sum14/1 -> Sum5/1
  Constant7/1 -> IF_INTER7/1(Z_i)
  IF_INTER6/1(y) -> CHK_CHAPP3/1(y)
  CHAPP_INTER3/1(y) -> Sum2/1, Scope1/1
  Constant4/1 -> CHAPP_INTER4/1(Z_i)
  TH1_i2/1 -> CHAPP_INTER3/2(Z)
  y3/1 -> Saturation3/1
  Constant5/1 -> IF_INTER5/1(Z_i)
  Sum13/1 -> Sum14/1
  Constant6/1 -> IF_INTER6/1(Z_i)

== system Full_model/TRAJECTORY_PLANNING/TH3_Interpolation/DELAY_IF16 ==
  In1 : Inport
  Constant : Constant  Value=0
  Constant52 : Constant  Value=0
  Ramp : simulink/Sources/Ramp  slope=1  start=0  InitialOutput=-(time_ri+time_ch_app+time_if+(2*time_plug)+ch_cyc)
  Ramp7 : simulink/Sources/Ramp  slope=1  start=0  InitialOutput=-(time_ri+time_ch_app+time_if)
  Switch1 : Switch  Criteria=u2 > Threshold
  Switch22 : Switch  Criteria=u2 > Threshold
  TH1 : Outport
  wires:
  Ramp/1 -> Switch1/2
  Constant/1 -> Switch1/1
  Switch1/1 -> TH1/1
  Switch22/1 -> Switch1/3
  Constant52/1 -> Switch22/3
  Ramp7/1 -> Switch22/2
  In1/1 -> Switch22/1

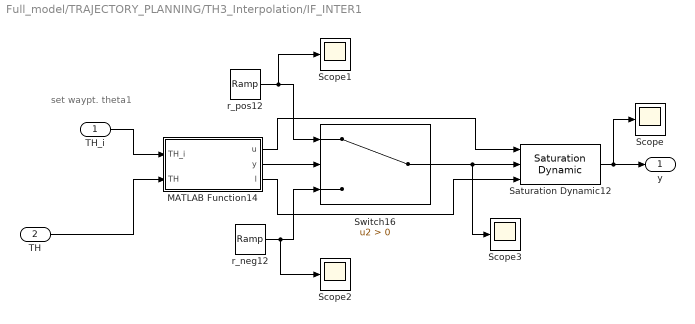
== system Full_model/TRAJECTORY_PLANNING/TH3_Interpolation/IF_INTER1 ==
  note: set waypt. theta1
  TH_i : Inport
  TH : Inport  Port=2
  MATLAB Function14 : MATLAB Function  TreatAsAtomicUnit=on
  Saturation Dynamic12 : simulink/Discontinuities/Saturation Dynamic  OutMin=[]  OutMax=[]  OutDataTypeStr=Inherit: Same as second input  OutDataType=fixdt(1, 16)  OutScaling=2^-10  DoSatur=off
  Scope{,1..3} (4 alike) : Scope
  Switch16 : Switch  Criteria=u2 > Threshold
  r_neg12 : simulink/Sources/Ramp  slope=-max_avel  start=time_ri  InitialOutput=0
  r_pos12 : simulink/Sources/Ramp  slope=max_avel  start=time_ri  InitialOutput=0
  y : Outport
  wires:
  TH_i/1 -> MATLAB Function14/1(TH_i)
  TH/1 -> MATLAB Function14/2(TH)
  r_pos12/1 -> Scope1/1, Switch16/1
  r_neg12/1 -> Scope2/1, Switch16/3
  Switch16/1 -> Saturation Dynamic12/2, Scope3/1
  MATLAB Function14/1(u) -> Saturation Dynamic12/1
  MATLAB Function14/2(y) -> Switch16/2
  MATLAB Function14/3(l) -> Saturation Dynamic12/3
  Saturation Dynamic12/1 -> Scope/1, y/1

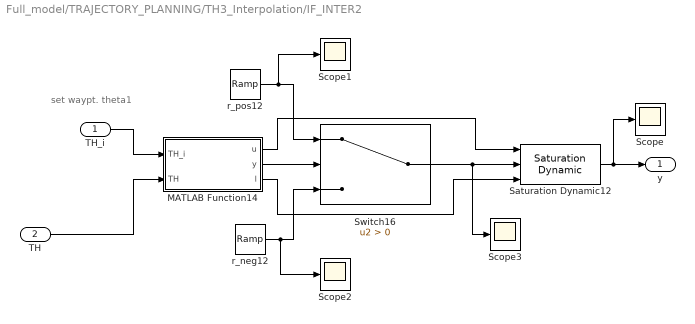
== system Full_model/TRAJECTORY_PLANNING/TH3_Interpolation/IF_INTER2 ==
  note: set waypt. theta1
  TH_i : Inport
  TH : Inport  Port=2
  MATLAB Function14 : MATLAB Function  TreatAsAtomicUnit=on
  Saturation Dynamic12 : simulink/Discontinuities/Saturation Dynamic  OutMin=[]  OutMax=[]  OutDataTypeStr=Inherit: Same as second input  OutDataType=fixdt(1, 16)  OutScaling=2^-10  DoSatur=off
  Scope{,1..3} (4 alike) : Scope
  Switch16 : Switch  Criteria=u2 > Threshold
  r_neg12 : simulink/Sources/Ramp  slope=-max_avel  start=(time_ri+time_ch_app+time_if+(2*time_plug)+ch_cyc)  InitialOutput=0
  r_pos12 : simulink/Sources/Ramp  slope=max_avel  start=(time_ri+time_ch_app+time_if+(2*time_plug)+ch_cyc)  InitialOutput=0
  y : Outport
  wires:
  Saturation Dynamic12/1 -> y/1, Scope/1
  MATLAB Function14/3(l) -> Saturation Dynamic12/3
  MATLAB Function14/2(y) -> Switch16/2
  MATLAB Function14/1(u) -> Saturation Dynamic12/1
  Switch16/1 -> Scope3/1, Saturation Dynamic12/2
  r_neg12/1 -> Switch16/3, Scope2/1
  r_pos12/1 -> Switch16/1, Scope1/1
  TH/1 -> MATLAB Function14/2(TH)
  TH_i/1 -> MATLAB Function14/1(TH_i)

== system Full_model/TRAJECTORY_PLANNING/TH3_Interpolation/IF_INTER3 ==
  note: set waypt. theta1
  TH_i : Inport
  TH : Inport  Port=2
  MATLAB Function14 : MATLAB Function  TreatAsAtomicUnit=on
  Saturation Dynamic12 : simulink/Discontinuities/Saturation Dynamic  OutMin=[]  OutMax=[]  OutDataTypeStr=Inherit: Same as second input  OutDataType=fixdt(1, 16)  OutScaling=2^-10  DoSatur=off
  Scope{,1..3} (4 alike) : Scope
  Switch16 : Switch  Criteria=u2 > Threshold
  r_neg12 : simulink/Sources/Ramp  slope=-max_avel  start=0  InitialOutput=TH3_ri-(TH1_ri+TH2_ri)
  r_pos12 : simulink/Sources/Ramp  slope=max_avel  start=0  InitialOutput=TH3_ri-(TH1_ri+TH2_ri)
  y : Outport
  wires:
  Saturation Dynamic12/1 -> y/1, Scope/1
  MATLAB Function14/3(l) -> Saturation Dynamic12/3
  MATLAB Function14/2(y) -> Switch16/2
  MATLAB Function14/1(u) -> Saturation Dynamic12/1
  Switch16/1 -> Scope3/1, Saturation Dynamic12/2
  r_neg12/1 -> Switch16/3, Scope2/1
  r_pos12/1 -> Switch16/1, Scope1/1
  TH/1 -> MATLAB Function14/2(TH)
  TH_i/1 -> MATLAB Function14/1(TH_i)

== system Full_model/TRAJECTORY_PLANNING/TH4_Interpolation/IF_INTER1 ==
  note: set waypt. theta1
  TH_i : Inport
  TH : Inport  Port=2
  MATLAB Function14 : MATLAB Function  TreatAsAtomicUnit=on
  Saturation Dynamic12 : simulink/Discontinuities/Saturation Dynamic  OutMin=[]  OutMax=[]  OutDataTypeStr=Inherit: Same as second input  OutDataType=fixdt(1, 16)  OutScaling=2^-10  DoSatur=off
  Scope{,1..3} (4 alike) : Scope
  Switch16 : Switch  Criteria=u2 > Threshold
  r_neg12 : simulink/Sources/Ramp  slope=-max_avel  start=time_ri  InitialOutput=0
  r_pos12 : simulink/Sources/Ramp  slope=max_avel  start=time_ri  InitialOutput=0
  y : Outport
  wires:
  TH_i/1 -> MATLAB Function14/1(TH_i)
  TH/1 -> MATLAB Function14/2(TH)
  r_pos12/1 -> Scope1/1, Switch16/1
  r_neg12/1 -> Scope2/1, Switch16/3
  Switch16/1 -> Saturation Dynamic12/2, Scope3/1
  MATLAB Function14/1(u) -> Saturation Dynamic12/1
  MATLAB Function14/2(y) -> Switch16/2
  MATLAB Function14/3(l) -> Saturation Dynamic12/3
  Saturation Dynamic12/1 -> Scope/1, y/1

== system Full_model/TRAJECTORY_PLANNING/TH4_Interpolation/IF_INTER2 ==
  note: set waypt. theta1
  TH_i : Inport
  TH : Inport  Port=2
  MATLAB Function14 : MATLAB Function  TreatAsAtomicUnit=on
  Saturation Dynamic12 : simulink/Discontinuities/Saturation Dynamic  OutMin=[]  OutMax=[]  OutDataTypeStr=Inherit: Same as second input  OutDataType=fixdt(1, 16)  OutScaling=2^-10  DoSatur=off
  Scope{,1..3} (4 alike) : Scope
  Switch16 : Switch  Criteria=u2 > Threshold
  r_neg12 : simulink/Sources/Ramp  slope=-max_avel  start=(time_ri+time_ch_app+time_if+(2*time_plug)+ch_cyc)  InitialOutput=0
  r_pos12 : simulink/Sources/Ramp  slope=max_avel  start=(time_ri+time_ch_app+time_if+(2*time_plug)+ch_cyc)  InitialOutput=0
  y : Outport
  wires:
  Saturation Dynamic12/1 -> y/1, Scope/1
  MATLAB Function14/3(l) -> Saturation Dynamic12/3
  MATLAB Function14/2(y) -> Switch16/2
  MATLAB Function14/1(u) -> Saturation Dynamic12/1
  Switch16/1 -> Scope3/1, Saturation Dynamic12/2
  r_neg12/1 -> Switch16/3, Scope2/1
  r_pos12/1 -> Switch16/1, Scope1/1
  TH/1 -> MATLAB Function14/2(TH)
  TH_i/1 -> MATLAB Function14/1(TH_i)

== system Full_model/TRAJECTORY_PLANNING/TH4_Interpolation/IF_INTER5 ==
  note: set waypt. theta1
  TH_i : Inport
  TH : Inport  Port=2
  MATLAB Function14 : MATLAB Function  TreatAsAtomicUnit=on
  Saturation Dynamic12 : simulink/Discontinuities/Saturation Dynamic  OutMin=[]  OutMax=[]  OutDataTypeStr=Inherit: Same as second input  OutDataType=fixdt(1, 16)  OutScaling=2^-10  DoSatur=off
  Scope{,1..3} (4 alike) : Scope
  Switch16 : Switch  Criteria=u2 > Threshold
  r_neg12 : simulink/Sources/Ramp  slope=-max_avel  start=0  InitialOutput=TH4_ri
  r_pos12 : simulink/Sources/Ramp  slope=max_avel  start=0  InitialOutput=TH4_ri
  y : Outport
  wires:
  Saturation Dynamic12/1 -> y/1, Scope/1
  MATLAB Function14/3(l) -> Saturation Dynamic12/3
  MATLAB Function14/2(y) -> Switch16/2
  MATLAB Function14/1(u) -> Saturation Dynamic12/1
  Switch16/1 -> Scope3/1, Saturation Dynamic12/2
  r_neg12/1 -> Switch16/3, Scope2/1
  r_pos12/1 -> Switch16/1, Scope1/1
  TH/1 -> MATLAB Function14/2(TH)
  TH_i/1 -> MATLAB Function14/1(TH_i)

== system Full_model/TRAJECTORY_PLANNING/TS_JA_Interpolation/DELAY_IF16 ==
  In1 : Inport
  Constant52 : Constant  Value=0
  Ramp7 : simulink/Sources/Ramp  slope=1  start=0  InitialOutput=-(time_ri+time_ch_app+time_if)
  Switch22 : Switch  Criteria=u2 > Threshold
  TH1 : Outport
  wires:
  Switch22/1 -> TH1/1
  Constant52/1 -> Switch22/3
  Ramp7/1 -> Switch22/2
  In1/1 -> Switch22/1

== system Full_model/TRAJECTORY_PLANNING/TS_JA_Interpolation/DELAY_IF17 ==
  In1 : Inport
  Constant52 : Constant  Value=0
  Ramp7 : simulink/Sources/Ramp  slope=1  start=0  InitialOutput=-(time_ri+time_ch_app+time_if)
  Switch22 : Switch  Criteria=u2 > Threshold
  TH2 : Outport
  wires:
  In1/1 -> Switch22/1
  Ramp7/1 -> Switch22/2
  Constant52/1 -> Switch22/3
  Switch22/1 -> TH2/1

== system Full_model/TRAJECTORY_PLANNING/TS_JA_Interpolation/IK_BLOCK1 ==
  XE : Inport
  YE : Inport  Port=2
  Constant : Constant  Value=l_app
  Constant1 : Constant  Value=L1
  Constant2 : Constant  Value=L2
  MATLAB Function : MATLAB Function  TreatAsAtomicUnit=on
  TH1_1 : MATLAB Function  TreatAsAtomicUnit=on
  TH1_2 : MATLAB Function  TreatAsAtomicUnit=on
  TH2_1 : MATLAB Function  TreatAsAtomicUnit=on
  TH2_2 : MATLAB Function  TreatAsAtomicUnit=on
  TH1 : Outport
  TH2 : Outport  Port=2
  wires:
  MATLAB Function/2(TH2) -> TH2/1
  MATLAB Function/1(TH1) -> TH1/1
  TH2_1/1(out1) -> MATLAB Function/4(TH2_1)
  TH2_2/1(out1) -> MATLAB Function/3(TH2_2)
  TH1_2/1(out1) -> MATLAB Function/2(TH1_2)
  TH1_1/1(out1) -> MATLAB Function/1(TH1_1)
  YE/1 -> TH2_2/4(YE), TH1_1/4(YE), TH1_2/4(YE), TH2_1/4(YE)
  XE/1 -> TH2_2/3(XE), TH2_1/3(XE), TH1_1/3(XE), TH1_2/3(XE)
  Constant2/1 -> TH1_2/2(L_2), TH2_2/2(L_2), TH2_1/2(L_2), TH1_1/2(L_2)
  Constant1/1 -> TH1_1/1(L_1), TH1_2/1(L_1), TH2_2/1(L_1), TH2_1/1(L_1)
  Constant/1 -> MATLAB Function/5(l_app)

== system Full_model/TRAJECTORY_PLANNING/TS_JA_Interpolation/X_Plug-in_TS_Interpolation ==
  Constant8 : Constant  Value=L2xf
  Ramp : simulink/Sources/Ramp  slope=xp_vel  start=(time_ri+time_ch_app+time_if)  InitialOutput=0
  Saturation2 : Saturate  UpperLimit=max(xp_dist,-xp_dist)  LowerLimit=min(xp_dist,-xp_dist)
  Saturation5 : Saturate  UpperLimit=max(xp_dist,-xp_dist)  LowerLimit=min(xp_dist,-xp_dist)
  Sum15 : Sum  Inputs=|+-
  Sum9 : Sum  Inputs=|++
  y5 : simulink/Sources/Ramp  slope=xp_vel  start=(time_ri+time_ch_app+time_if+time_plug+ch_cyc)  InitialOutput=0
  X_TS : Outport
  wires:
  Saturation5/1 -> Sum15/2
  Constant8/1 -> Sum9/2
  Saturation2/1 -> Sum9/1
  Sum15/1 -> X_TS/1
  Sum9/1 -> Sum15/1
  y5/1 -> Saturation5/1
  Ramp/1 -> Saturation2/1

== system Full_model/TRAJECTORY_PLANNING/TS_JA_Interpolation/Y_Plug-in_TS_Interpolation ==
  Constant9 : Constant  Value=L2yf
  Saturation1 : Saturate  UpperLimit=max(yp_dist,-yp_dist)  LowerLimit=min(yp_dist,-yp_dist)
  Saturation6 : Saturate  UpperLimit=max(yp_dist,-yp_dist)  LowerLimit=min(yp_dist,-yp_dist)
  Sum10 : Sum  Inputs=|++
  Sum16 : Sum  Inputs=|+-
  y2 : simulink/Sources/Ramp  slope=yp_vel  start=(time_ri+time_ch_app+time_if)  InitialOutput=0
  y6 : simulink/Sources/Ramp  slope=yp_vel  start=(time_ri+time_ch_app+time_if+time_plug+ch_cyc)  InitialOutput=0
  Y_TS : Outport
  wires:
  y6/1 -> Saturation6/1
  Saturation1/1 -> Sum10/1
  Sum10/1 -> Sum16/1
  Constant9/1 -> Sum10/2
  Saturation6/1 -> Sum16/2
  y2/1 -> Saturation1/1
  Sum16/1 -> Y_TS/1

== system Full_model/TRAJECTORY_PLANNING/Z_Interpolation/CHAPP_INTER3 ==
  Z_i : Inport
  Z : Inport  Port=2
  MATLAB Function12 : MATLAB Function  TreatAsAtomicUnit=on
  Saturation Dynamic10 : simulink/Discontinuities/Saturation Dynamic  OutMin=[]  OutMax=[]  OutDataTypeStr=Inherit: Same as second input  OutDataType=fixdt(1, 16)  OutScaling=2^-10  DoSatur=off
  Switch14 : Switch  Criteria=u2 > Threshold
  r_neg10 : simulink/Sources/Ramp  slope=-max_tvel  start=time_ri_ang  InitialOutput=L2rz
  r_pos10 : simulink/Sources/Ramp  slope=max_tvel  start=time_ri_ang  InitialOutput=L2rz
  y : Outport
  wires:
  Z_i/1 -> MATLAB Function12/1(Z_i)
  MATLAB Function12/3(l) -> Saturation Dynamic10/3
  Saturation Dynamic10/1 -> y/1
  Z/1 -> MATLAB Function12/2(Z)
  r_pos10/1 -> Switch14/1
  MATLAB Function12/2(y) -> Switch14/2
  Switch14/1 -> Saturation Dynamic10/2
  r_neg10/1 -> Switch14/3
  MATLAB Function12/1(u) -> Saturation Dynamic10/1

== system Full_model/TRAJECTORY_PLANNING/Z_Interpolation/CHAPP_INTER4 ==
  Z_i : Inport
  Z : Inport  Port=2
  MATLAB Function12 : MATLAB Function  TreatAsAtomicUnit=on
  Saturation Dynamic10 : simulink/Discontinuities/Saturation Dynamic  OutMin=[]  OutMax=[]  OutDataTypeStr=Inherit: Same as second input  OutDataType=fixdt(1, 16)  OutScaling=2^-10  DoSatur=off
  Switch14 : Switch  Criteria=u2 > Threshold
  r_neg10 : simulink/Sources/Ramp  slope=-max_tvel  start=time_ri  InitialOutput=0
  r_pos10 : simulink/Sources/Ramp  slope=max_tvel  start=time_ri  InitialOutput=0
  y : Outport
  wires:
  MATLAB Function12/1(u) -> Saturation Dynamic10/1
  r_neg10/1 -> Switch14/3
  Switch14/1 -> Saturation Dynamic10/2
  MATLAB Function12/2(y) -> Switch14/2
  r_pos10/1 -> Switch14/1
  Z/1 -> MATLAB Function12/2(zpf)
  Saturation Dynamic10/1 -> y/1
  MATLAB Function12/3(l) -> Saturation Dynamic10/3
  Z_i/1 -> MATLAB Function12/1(Z_i)

== system Full_model/TRAJECTORY_PLANNING/Z_Interpolation/CHK_CHAPP3 ==
  y : Inport
  Constant46 : Constant  Value=-ch_app
  Constant49 : Constant  Value=0
  Switch19 : Switch  Criteria=u2 > Threshold
  Out1 : Outport
  wires:
  Constant46/1 -> Switch19/2
  Constant49/1 -> Switch19/3
  y/1 -> Switch19/1
  Switch19/1 -> Out1/1

== system Full_model/TRAJECTORY_PLANNING/Z_Interpolation/CHK_CHAPP4 ==
  y : Inport
  Constant46 : Constant  Value=ch_app
  Constant49 : Constant  Value=0
  Switch19 : Switch  Criteria=u2 > Threshold
  Out1 : Outport
  wires:
  Switch19/1 -> Out1/1
  y/1 -> Switch19/1
  Constant49/1 -> Switch19/3
  Constant46/1 -> Switch19/2

== system Full_model/TRAJECTORY_PLANNING/Z_Interpolation/CHK_CHAPP5 ==
  y : Inport
  Constant46 : Constant  Value=ch_app
  Constant49 : Constant  Value=0
  Switch19 : Switch  Criteria=u2 > Threshold
  Out1 : Outport
  wires:
  Switch19/1 -> Out1/1
  y/1 -> Switch19/1
  Constant49/1 -> Switch19/3
  Constant46/1 -> Switch19/2
